simulink library "base_lib"  (R2020b)
settings: Solver=VariableStepAuto  StartTime=0.0  StopTime=10.0  RelTol=1e-3
(part 1 of 2)
settings Model: Creator=maxjo65  LastModifiedBy=Max

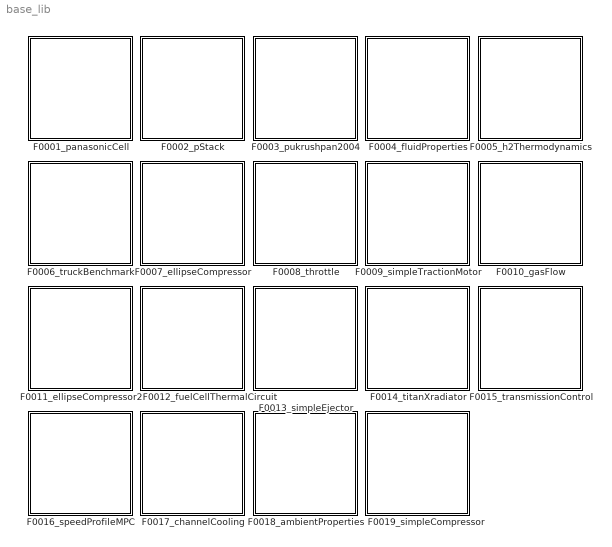
== system base_lib ==
  F0001_panasonicCell : Subsystem
  F0002_pStack : Subsystem
  F0003_pukrushpan2004 : Subsystem
  F0004_fluidProperties : Subsystem
  F0005_h2Thermodynamics : Subsystem
  F0006_truckBenchmark : Subsystem
  F0007_ellipseCompressor : Subsystem
  F0008_throttle : Subsystem
  F0009_simpleTractionMotor : Subsystem
  F0010_gasFlow : Subsystem
  F0011_ellipseCompressor2 : Subsystem
  F0012_fuelCellThermalCircuit : Subsystem
  F0013_simpleEjector : Subsystem
  F0014_titanXradiator : Subsystem
  F0015_transmissionControl : Subsystem
  F0016_speedProfileMPC : Subsystem
  F0017_channelCooling : Subsystem
  F0018_ambientProperties : Subsystem
  F0019_simpleCompressor : Subsystem

== system base_lib/F0001_panasonicCell ==
  F0001_cellCapacity.m : MATLAB Function  TreatAsAtomicUnit=on
  F0001_dynamicVoltage.m : MATLAB Function  TreatAsAtomicUnit=on
  F0001_ocvSOC.m : MATLAB Function  TreatAsAtomicUnit=on

== system base_lib/F0002_pStack ==
  F0002_pStackVoltage.m : MATLAB Function  TreatAsAtomicUnit=on

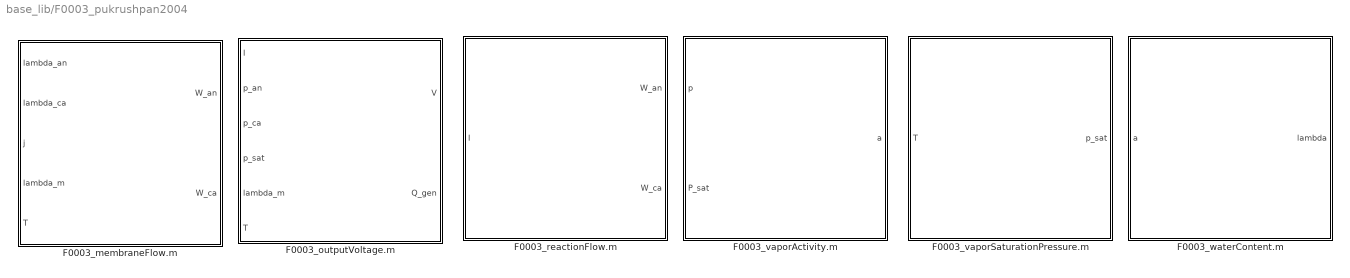
== system base_lib/F0003_pukrushpan2004 ==
  F0003_membraneFlow.m : MATLAB Function  TreatAsAtomicUnit=on
  F0003_outputVoltage.m : MATLAB Function  TreatAsAtomicUnit=on
  F0003_reactionFlow.m : MATLAB Function  TreatAsAtomicUnit=on
  F0003_vaporActivity.m : MATLAB Function  TreatAsAtomicUnit=on
  F0003_vaporSaturationPressure.m : MATLAB Function  TreatAsAtomicUnit=on
  F0003_waterContent.m : MATLAB Function  TreatAsAtomicUnit=on

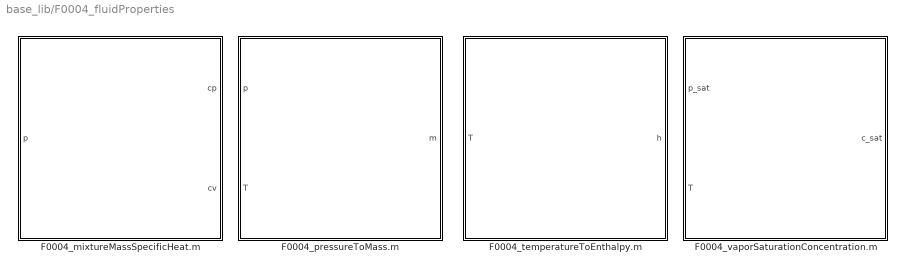
== system base_lib/F0004_fluidProperties ==
  F0004_mixtureMassSpecificHeat.m : MATLAB Function  TreatAsAtomicUnit=on
  F0004_pressureToMass.m : MATLAB Function  TreatAsAtomicUnit=on
  F0004_temperatureToEnthalpy.m : MATLAB Function  TreatAsAtomicUnit=on
  F0004_vaporSaturationConcentration.m : MATLAB Function  TreatAsAtomicUnit=on

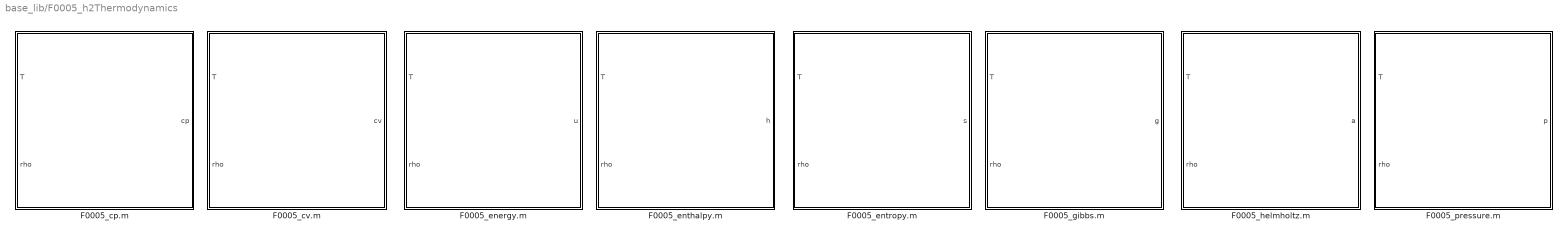
== system base_lib/F0005_h2Thermodynamics ==
  F0005_cp.m : MATLAB Function  TreatAsAtomicUnit=on
  F0005_cv.m : MATLAB Function  TreatAsAtomicUnit=on
  F0005_energy.m : MATLAB Function  TreatAsAtomicUnit=on
  F0005_enthalpy.m : MATLAB Function  TreatAsAtomicUnit=on
  F0005_entropy.m : MATLAB Function  TreatAsAtomicUnit=on
  F0005_gibbs.m : MATLAB Function  TreatAsAtomicUnit=on
  F0005_helmholtz.m : MATLAB Function  TreatAsAtomicUnit=on
  F0005_pressure.m : MATLAB Function  TreatAsAtomicUnit=on

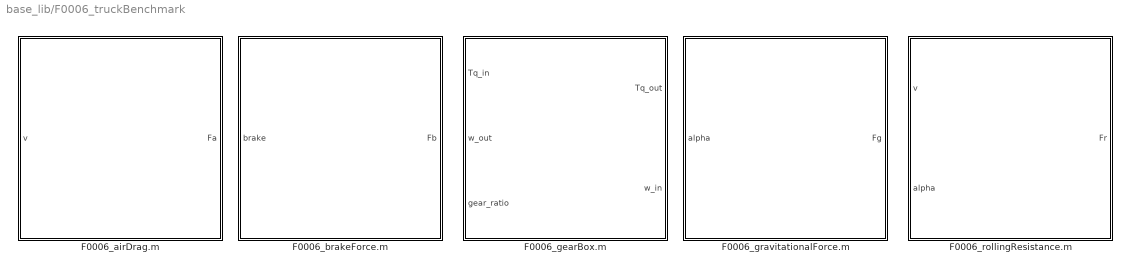
== system base_lib/F0006_truckBenchmark ==
  F0006_airDrag.m : MATLAB Function  TreatAsAtomicUnit=on
  F0006_brakeForce.m : MATLAB Function  TreatAsAtomicUnit=on
  F0006_gearBox.m : MATLAB Function  TreatAsAtomicUnit=on
  F0006_gravitationalForce.m : MATLAB Function  TreatAsAtomicUnit=on
  F0006_rollingResistance.m : MATLAB Function  TreatAsAtomicUnit=on

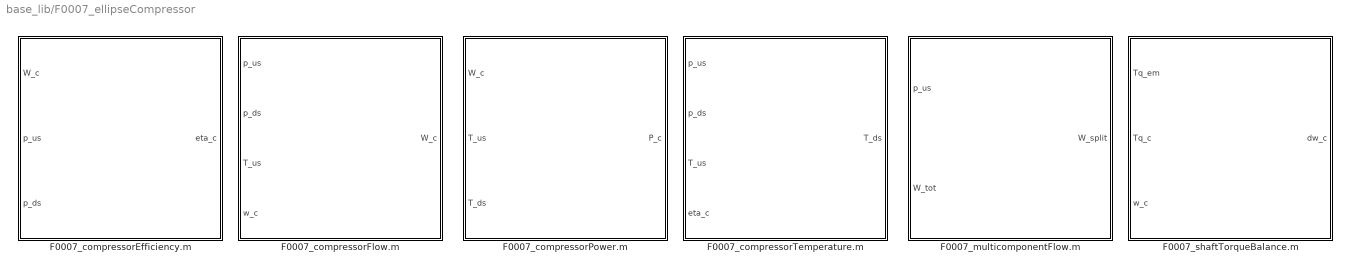
== system base_lib/F0007_ellipseCompressor ==
  F0007_compressorEfficiency.m : MATLAB Function  TreatAsAtomicUnit=on
  F0007_compressorFlow.m : MATLAB Function  TreatAsAtomicUnit=on
  F0007_compressorPower.m : MATLAB Function  TreatAsAtomicUnit=on
  F0007_compressorTemperature.m : MATLAB Function  TreatAsAtomicUnit=on
  F0007_multicomponentFlow.m : MATLAB Function  TreatAsAtomicUnit=on
  F0007_shaftTorqueBalance.m : MATLAB Function  TreatAsAtomicUnit=on

== system base_lib/F0008_throttle ==
  F0008_throttleFlow.m : MATLAB Function  TreatAsAtomicUnit=on
  F0008_throttleFlow2.m : MATLAB Function  TreatAsAtomicUnit=on

== system base_lib/F0009_simpleTractionMotor ==
  F0009_currentDemand.m : MATLAB Function  TreatAsAtomicUnit=on
  F0009_torqueLimit.m : MATLAB Function  TreatAsAtomicUnit=on

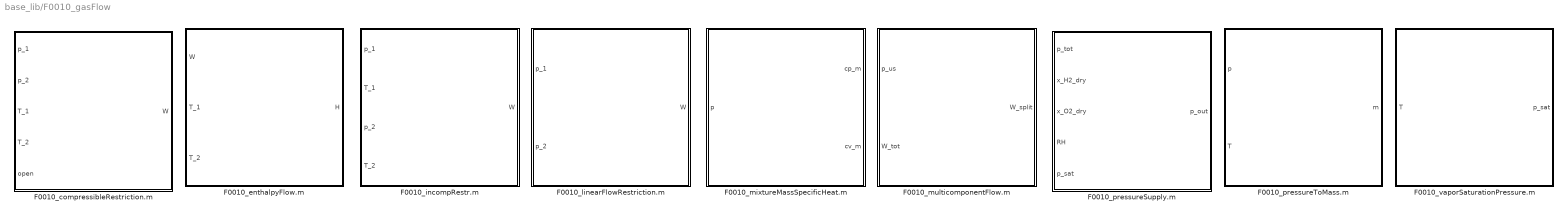
== system base_lib/F0010_gasFlow ==
  F0010_compressibleRestriction.m : MATLAB Function  TreatAsAtomicUnit=on
  F0010_enthalpyFlow.m : MATLAB Function  TreatAsAtomicUnit=on
  F0010_incompRestr.m : MATLAB Function  TreatAsAtomicUnit=on
  F0010_linearFlowRestriction.m : MATLAB Function  TreatAsAtomicUnit=on
  F0010_mixtureMassSpecificHeat.m : MATLAB Function  TreatAsAtomicUnit=on
  F0010_multicomponentFlow.m : MATLAB Function  TreatAsAtomicUnit=on
  F0010_pressureSupply.m : MATLAB Function  TreatAsAtomicUnit=on
  F0010_pressureToMass.m : MATLAB Function  TreatAsAtomicUnit=on
  F0010_vaporSaturationPressure.m : MATLAB Function  TreatAsAtomicUnit=on

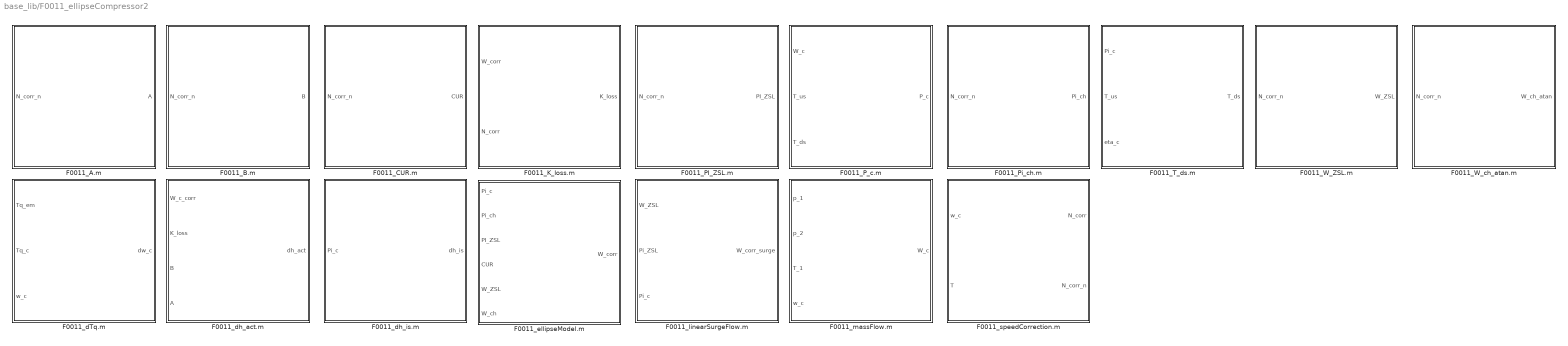
== system base_lib/F0011_ellipseCompressor2 ==
  F0011_A.m : MATLAB Function  TreatAsAtomicUnit=on
  F0011_B.m : MATLAB Function  TreatAsAtomicUnit=on
  F0011_CUR.m : MATLAB Function  TreatAsAtomicUnit=on
  F0011_K_loss.m : MATLAB Function  TreatAsAtomicUnit=on
  F0011_PI_ZSL.m : MATLAB Function  TreatAsAtomicUnit=on
  F0011_P_c.m : MATLAB Function  TreatAsAtomicUnit=on
  F0011_Pi_ch.m : MATLAB Function  TreatAsAtomicUnit=on
  F0011_T_ds.m : MATLAB Function  TreatAsAtomicUnit=on
  F0011_W_ZSL.m : MATLAB Function  TreatAsAtomicUnit=on
  F0011_W_ch_atan.m : MATLAB Function  TreatAsAtomicUnit=on
  F0011_dTq.m : MATLAB Function  TreatAsAtomicUnit=on
  F0011_dh_act.m : MATLAB Function  TreatAsAtomicUnit=on
  F0011_dh_is.m : MATLAB Function  TreatAsAtomicUnit=on
  F0011_ellipseModel.m : MATLAB Function  TreatAsAtomicUnit=on
  F0011_linearSurgeFlow.m : MATLAB Function  TreatAsAtomicUnit=on
  F0011_massFlow.m : MATLAB Function  TreatAsAtomicUnit=on
  F0011_speedCorrection.m : MATLAB Function  TreatAsAtomicUnit=on

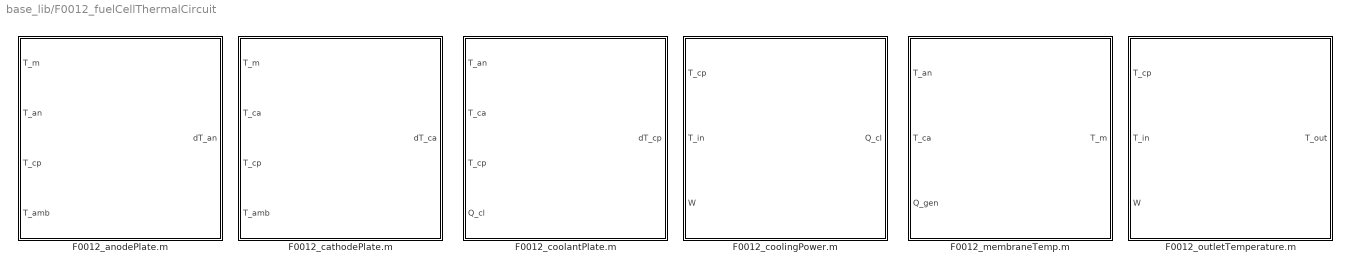
== system base_lib/F0012_fuelCellThermalCircuit ==
  F0012_anodePlate.m : MATLAB Function  TreatAsAtomicUnit=on
  F0012_cathodePlate.m : MATLAB Function  TreatAsAtomicUnit=on
  F0012_coolantPlate.m : MATLAB Function  TreatAsAtomicUnit=on
  F0012_coolingPower.m : MATLAB Function  TreatAsAtomicUnit=on
  F0012_membraneTemp.m : MATLAB Function  TreatAsAtomicUnit=on
  F0012_outletTemperature.m : MATLAB Function  TreatAsAtomicUnit=on

== system base_lib/F0013_simpleEjector ==
  F0013_ejectorModel.m : MATLAB Function  TreatAsAtomicUnit=on

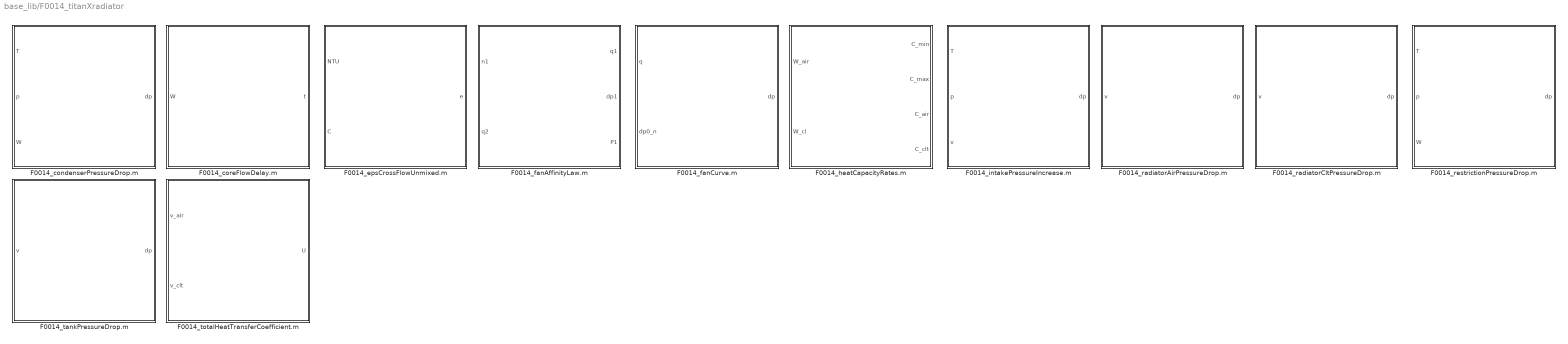
== system base_lib/F0014_titanXradiator ==
  F0014_condenserPressureDrop.m : MATLAB Function  TreatAsAtomicUnit=on
  F0014_coreFlowDelay.m : MATLAB Function  TreatAsAtomicUnit=on
  F0014_epsCrossFlowUnmixed.m : MATLAB Function  TreatAsAtomicUnit=on
  F0014_fanAffinityLaw.m : MATLAB Function  TreatAsAtomicUnit=on
  F0014_fanCurve.m : MATLAB Function  TreatAsAtomicUnit=on
  F0014_heatCapacityRates.m : MATLAB Function  TreatAsAtomicUnit=on
  F0014_intakePressureIncrease.m : MATLAB Function  TreatAsAtomicUnit=on
  F0014_radiatorAirPressureDrop.m : MATLAB Function  TreatAsAtomicUnit=on
  F0014_radiatorCltPressureDrop.m : MATLAB Function  TreatAsAtomicUnit=on
  F0014_restrictionPressureDrop.m : MATLAB Function  TreatAsAtomicUnit=on
  F0014_tankPressureDrop.m : MATLAB Function  TreatAsAtomicUnit=on
  F0014_totalHeatTransferCoefficient.m : MATLAB Function  TreatAsAtomicUnit=on

== system base_lib/F0015_transmissionControl ==
  F0015_gearSelector.m : MATLAB Function  TreatAsAtomicUnit=on
  F0015_transmissionControlUnit.m : MATLAB Function  TreatAsAtomicUnit=on

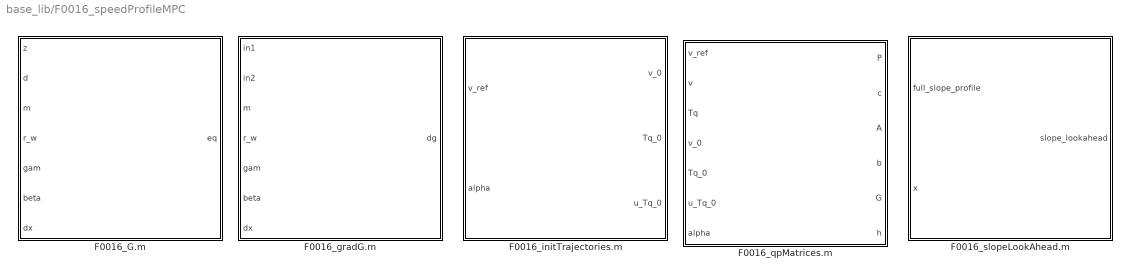
== system base_lib/F0016_speedProfileMPC ==
  F0016_G.m : MATLAB Function  TreatAsAtomicUnit=on
  F0016_gradG.m : MATLAB Function  TreatAsAtomicUnit=on
  F0016_initTrajectories.m : MATLAB Function  TreatAsAtomicUnit=on
  F0016_qpMatrices.m : MATLAB Function  TreatAsAtomicUnit=on
  F0016_slopeLookAhead.m : MATLAB Function  TreatAsAtomicUnit=on

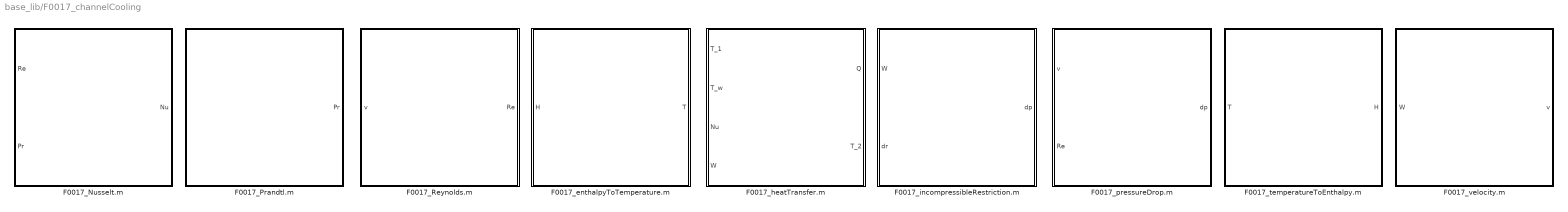
== system base_lib/F0017_channelCooling ==
  F0017_Nusselt.m : MATLAB Function  TreatAsAtomicUnit=on
  F0017_Prandtl.m : MATLAB Function  TreatAsAtomicUnit=on
  F0017_Reynolds.m : MATLAB Function  TreatAsAtomicUnit=on
  F0017_enthalpyToTemperature.m : MATLAB Function  TreatAsAtomicUnit=on
  F0017_heatTransfer.m : MATLAB Function  TreatAsAtomicUnit=on
  F0017_incompressibleRestriction.m : MATLAB Function  TreatAsAtomicUnit=on
  F0017_pressureDrop.m : MATLAB Function  TreatAsAtomicUnit=on
  F0017_temperatureToEnthalpy.m : MATLAB Function  TreatAsAtomicUnit=on
  F0017_velocity.m : MATLAB Function  TreatAsAtomicUnit=on

== system base_lib/F0018_ambientProperties ==
  F0018_troposphereModel.m : MATLAB Function  TreatAsAtomicUnit=on

== system base_lib/F0019_simpleCompressor ==
  F0007_compressorPower.m : MATLAB Function  TreatAsAtomicUnit=on
  F0007_compressorTemperature.m : MATLAB Function  TreatAsAtomicUnit=on
  F0007_multicomponentFlow.m : MATLAB Function  TreatAsAtomicUnit=on

== matlab function base_lib/F0003_pukrushpan2004/F0003_waterContent.m ==
  data: a input; lambda output
function lambda = F0003_waterContent(a)
lambda = zeros(length(a),1);
lambda( a <= 1) = 0.043 + 17.81.*a - 39.85.*a.^2 + 36.*a.^3;
lambda( a > 1)  = 14 + 1.4*(a-1);
end

== matlab function base_lib/F0004_fluidProperties/F0004_mixtureMassSpecificHeat.m ==
  data: p input; cp output; cv output; par parameter
function [cp, cv] = F0004_mixtureMassSpecificHeat(p, par)
% total pressure
p_tot = sum(p);

% mass specific heat capacity
cp_r  = par.cp_r;
cp_v  = par.cp_H2O;
cp_N2 = par.cp_N2;
R_r    = par.R_r;
R_H2O  = par.R_H2O;
R_N2   = par.R_N2;

% partial pressures
p_r  = p(1);
p_v  = p(2);
p_N2 = p(3);

% mole fractions
x_r   = p_r  ./ p_tot;
x_v   = p_v  ./ p_tot;
x_N2  = p_N2 ./ p_tot;

% average mass
M_avg = sum([x_r, x_v, x_N2] .* [par.M_r, par.M_H2O, par.M_N2]);

% mole fraction to mass fraction
w_r   = x_r  .* par.M_r   ./ M_avg;
w_v   = x_v  .* par.M_H2O ./ M_avg;
w_N2  = x_N2 .* par.M_N2  ./ M_avg;

% mixture gas constant
Rm = w_r.*R_r + w_v.*R_H2O + w_N2 .* R_N2;

% ideal mixture heat capacity
cp = w_r.*cp_r + w_v.*cp_v + w_N2 .* cp_N2;
cv = cp - Rm;

end

== matlab function base_lib/F0004_fluidProperties/F0004_pressureToMass.m ==
  data: p input; m output; T input; par parameter
function m = F0004_pressureToMass(p, T, par)
% gas constants
R_r    = par.R_r;
R_H2O  = par.R_H2O;
R_N2   = par.R_N2;
Rj     = [R_r; R_H2O; R_N2];
V      = par.V;

% mass
m = p .* V ./ (Rj .* T);
end

== matlab function base_lib/F0004_fluidProperties/F0004_temperatureToEnthalpy.m ==
  data: T input; h output; par parameter
function h = F0004_temperatureToEnthalpy(T, par)
% output size
h = zeros(3,1);

% mass heat capacity
cp_r  = par.cp_r;
cp_v  = par.cp_H2O;
cp_N2 = par.cp_N2;
cp    = [cp_r; cp_v; cp_N2];

% specific enthalpy
h = cp .* T;
end

== matlab function base_lib/F0004_fluidProperties/F0004_vaporSaturationConcentration.m ==
  data: p_sat input; c_sat output; T input; par parameter
function c_sat = F0004_vaporSaturationConcentration(p_sat, T, par)
% saturation concentration
c_sat = p_sat ./ (par.R .* T);

end

== matlab function base_lib/F0005_h2Thermodynamics/F0005_cp.m ==
  data: T input; cp output; rho input
function cp = F0005_cp(T,rho)
%ISOBARICHEATCAPACITY
%    CP = ISOBARICHEATCAPACITY(T,RHO)

%    This function was generated by the Symbolic Math Toolbox version 8.7.
%    04-Nov-2021 19:06:05

t2 = rho.^2;
t3 = rho.^3;
t4 = 1.0./T;
t5 = rho./1.5508e+4;
t9 = rho.*2.17307196285788e-4;
t10 = rho.*1.328346659788496e-5;
t11 = rho.*6.30642249161723e-5;
t12 = rho.*3.231880319834924e-4;
t13 = rho.*2.072478720660304e-4;
t6 = -t5;
t8 = t4.*3.3145e+1;
t14 = t5-3.9e+1./2.5e+2;
t15 = t5-6.7e+1./1.0e+2;
t16 = t5-2.17e+2./1.25e+2;
t17 = t4.*8.644216;
t18 = t4.*1.133559e+1;
t19 = t4.*1.4882105e+1;
t20 = t4.*1.8461765e+1;
t21 = t5-7.53e+2./5.0e+2;
t22 = t5-8.31e+2./5.0e+2;
t26 = t4.*2.6297243e+1;
t53 = t10-3.57616e-1;
t59 = t9-5.07522;
t60 = t11-1.52568e-1;
t61 = t12-3.35804;
t68 = t13-5.341668;
t69 = t3.*t4.*3.554762889834598e-13;
t92 = t4.*6.858999999999336e+3;
t94 = t4.*5.309999999993605e+2;
t95 = t4.*1.98899999999884e+3;
t97 = t4.*2.484000000001446e+3;
t98 = t4.*7.51000000000887e+2;
t7 = exp(t6);
t23 = t14.^2;
t24 = t15.^2;
t25 = t16.^2;
t27 = t8.^(3.77e+2./5.0e+2);
t28 = t21.^2;
t29 = t22.^2;
t30 = t8.^(3.11e+2./1.0e+3);
t31 = t8.^(8.77e+2./5.0e+2);
t32 = t8.^(4.89e+2./1.0e+3);
t33 = t8.^(9.93e+2./5.0e+2);
t34 = t8.^2.986;
t35 = t8.^4.646;
t36 = t8.^5.646;
t37 = 1.0./t8.^(2.09e+2./1.0e+3);
t38 = t8.^(7.91e+2./1.0e+3);
t39 = t8.^(8.03e+2./1.0e+3);
t40 = t8.^(9.89e+2./1.0e+3);
t41 = t8.^1.311;
t42 = t8.^1.409;
t43 = t8.^3.187;
t44 = t8.^6.844e-1;
t45 = t8.^4.187;
t46 = t8.^1.1444;
t47 = t8.^6.249;
t48 = t8.^7.249;
t49 = t8-7.164e-1;
t50 = t8-7.204e-1;
t51 = t8-1.5445;
t52 = t8-1.3444;
t54 = t8-1.4517;
t77 = t18-2.450088e-1;
t82 = t19-6.036356e-1;
t83 = t20-4.012628e-1;
t84 = t17-3.7860336e-1;
t90 = t26-1.2254063;
t96 = -t92;
t99 = -t94;
t100 = -t95;
t101 = -t97;
t102 = -t98;
t55 = t49.^2;
t56 = t50.^2;
t57 = t51.^2;
t58 = t52.^2;
t62 = t54.^2;
t63 = t23.*(4.89e+2./1.0e+3);
t64 = t25.*(1.03e+2./1.0e+3);
t66 = t28.*(3.37e+2./2.0e+2);
t67 = t24.*2.506;
t73 = t29.*1.607;
t78 = t40.*2.1101;
t91 = rho.*t46.*1.729249419654372e-4;
t103 = exp(t96);
t104 = exp(t99);
t105 = exp(t100);
t106 = exp(t101);
t107 = exp(t102);
t113 = t32.*4.52059;
t114 = t44.*6.93643;
t116 = rho.*t39.*9.447562548362136e-5;
t119 = t7.*t31.*7.77414e-1;
t126 = t2.*t42.*1.633921676808176e-9;
t129 = rho.*t7.*t31.*5.012986845499098e-5;
t131 = t2.*t7.*t41.*4.390189186720438e-9;
t132 = t3.*t7.*t41.*9.43639666993474e-14;
t65 = -t63;
t70 = -t64;
t71 = -t66;
t72 = -t67;
t74 = -t73;
t75 = t55.*(1.71e+2./1.0e+3);
t76 = t58.*2.245e-1;
t80 = t56.*2.785e-1;
t86 = t57.*3.967e-1;
t87 = t62.*1.304e-1;
t93 = -t91;
t108 = t103-1.0;
t109 = t104-1.0;
t110 = t105-1.0;
t111 = t106-1.0;
t112 = t107-1.0;
t115 = -t114;
t122 = -t119;
t133 = -t132;
t79 = -t75;
t81 = -t76;
t85 = -t80;
t88 = -t86;
t89 = -t87;
t117 = t65+t81;
t118 = t71+t79;
t121 = t72+t85;
t124 = t70+t89;
t128 = t74+t88;
t120 = exp(t117);
t123 = exp(t118);
t125 = exp(t121);
t127 = exp(t124);
t130 = exp(t128);
t134 = t36.*t120.*2.26312e-2;
t135 = t48.*t125.*2.31752e-2;
t137 = t34.*t130.*5.57346e-2;
t138 = rho.*t45.*t123.*2.730410110910498e-6;
t140 = t2.*t38.*t127.*4.015042715686892e-10;
t141 = rho.*t36.*t60.*t120.*1.459324219757545e-6;
t143 = rho.*t48.*t61.*t125.*1.494402888831571e-6;
t144 = rho.*t34.*t68.*t130.*3.593925715759608e-6;
t145 = t2.*t45.*t59.*t123.*8.803230948254119e-11;
t147 = t3.*t38.*t53.*t127.*8.630046246425269e-15;
t136 = -t135;
t139 = -t138;
t142 = -t141;
t146 = -t144;
t148 = -t147;
t149 = t69+t78+t93+t113+t115+t116+t122+t126+t129+t131+t133+t134+t136+t137+t139+t140+t142+t143+t145+t146+t148;
et1 = 1.0./t109.^2.*exp(t4.*(-1.061999999998721e+3)).*4.147575991701757e+2;
et2 = 1.0./t110.^2.*exp(t4.*(-3.977999999997681e+3)).*(-2.852060285124163e+3);
et3 = 1.0./t108.^2.*exp(t4.*(-1.371799999999867e+4)).*5.211660743085801e+4;
et4 = 1.0./t111.^2.*exp(t4.*(-4.968000000002893e+3)).*4.257320460091549e+3;
et5 = 1.0./t112.^2.*exp(t4.*(-1.502000000001774e+3)).*(-2.113609217775546e+2)+rho.*1.0./t8.^1.011.*1.480253927005417e-6;
et6 = rho.*1.0./t8.^1.511.*7.283985740327573e-5-rho.*1.0./t8.^1.3156.*9.661114093340211e-5-(t103.*5.211660743085801e+4)./t108;
et7 = (t104.*(-4.147575991701757e+2))./t109+(t105.*2.852060285124163e+3)./t110;
et8 = (t106.*(-4.257320460091549e+3))./t111+(t107.*2.113609217775546e+2)./t112;
et9 = t3.*1.0./t8.^(5.91e+2./1.0e+3).*(-2.023897381636773e-14)+t2.*1.0./t8.^1.197.*4.818543226360442e-10+t2.*1.0./t8.^8.556e-1.*9.213335645379665e-10;
et10 = 1.0./t4.^2.*1.365385267005982e-3+rho.*t7.*1.0./t8.^(1.23e+2./5.0e+2).*6.629755310962085e-5-rho.*t8.^(4.93e+2./5.0e+2).*t130.*2.131268390389476e-5;
et11 = rho.*t8.^3.646.*t120.*(-3.827999475491359e-5)+rho.*t8.^5.249.*t125.*6.769495795558421e-5;
et12 = t3.*t7.*1.0./t8.^(6.89e+2./1.0e+3).*(-3.847417086662462e-14)+t3.*1.0./t8.^1.209.*t127.*1.426710615412779e-15;
et13 = t2.*t8.^2.187.*t123.*1.174700408733436e-9+rho.*t36.*t120.*6.552365746711375e-7+rho.*t34.*t130.*2.851420662883673e-6;
et14 = rho.*t48.*t125.*(-8.323824090791849e-7)+t3.*t38.*t127.*2.25071606106771e-15-t2.*t45.*t123.*3.010704984302909e-11;
et15 = rho.*t35.*t82.*t120.*1.647868908950219e-5+rho.*t33.*t90.*t130.*2.146292437451638e-5-rho.*t47.*t83.*t125.*2.166585308228011e-5;
et16 = t2.*t43.*t77.*t123.*(-7.371825596068e-10)+t3.*t37.*t84.*t127.*1.365273316184478e-14-rho.*t36.*t82.^2.*t120.*1.459324219757545e-6;
et17 = rho.*t34.*t90.^2.*t130.*(-3.593925715759608e-6)+rho.*t48.*t83.^2.*t125.*1.494402888831571e-6+t2.*t45.*t77.^2.*t123.*8.803230948254119e-11-t3.*t38.*t84.^2.*t127.*8.630046246425269e-15;
et18 = t39.*1.465128-t46.*2.68172-t129+t132+rho.*t42.*5.067771472788238e-5+t2.*t4.*1.653817886866649e-8+t7.*t31.*1.554828-t45.*t123.*4.23432e-2+t53.*t147+t60.*t141+t68.*t144;
et19 = rho.*t7.*t41.*1.361661078153211e-4-rho.*t36.*t120.*1.427219086922879e-6-rho.*t34.*t130.*1.155087725045138e-5+rho.*t38.*t127.*1.245305648697446e-5;
et20 = rho.*t48.*t125.*7.489947278823833e-6-t2.*t7.*t41.*8.780378373440877e-9-t3.*t38.*t127.*1.777789526763605e-15;
et21 = t2.*t45.*t123.*2.966688829561638e-10-t36.*t60.*t120.*4.52624e-2-t34.*t68.*t130.*1.114692e-1+t48.*t61.*t125.*4.63504e-2;
et22 = rho.*t45.*t59.*t123.*5.460820221820995e-6-t2.*t38.*t53.*t127.*8.030085431373784e-10-rho.*t48.*t61.^2.*t125.*1.494402888831571e-6-t2.*t45.*t59.^2.*t123.*8.803230948254119e-11;
et23 = t3./9.32410994128e+13-t7.*t27.*1.363584156+t35.*t120.*1.277757552e-1+t33.*t130.*1.664235156e-1-t47.*t125.*1.679970248e-1+t77.*t138+t83.*t135;
et24 = t82.*t141+t84.*t147+t90.*t144+rho.*1.0./t8.^(1.97e+2./1.0e+3).*7.586392726334795e-5-rho.*t8.^1.444e-1.*1.978953035852463e-4+t2.*t8.^(4.09e+2./1.0e+3).*2.30219564262272e-9+1.0./t8.^(1.1e+1./1.0e+3).*2.0868889;
et25 = 1.0./t8.^(5.11e+2./1.0e+3).*2.21056851-1.0./t8.^3.156e-1.*4.747292692+rho.*t7.*t27.*8.792778927005417e-5-rho.*t43.*t123.*1.143222713438225e-5;
et26 = t2.*t7.*t30.*5.755538023790495e-9-t3.*t7.*t30.*1.237111603428444e-13+t2.*t37.*t127.*3.175898788108332e-10;
et27 = t36.*t82.*t120.*(-2.26312e-2)-t34.*t90.*t130.*5.57346e-2-rho.*t35.*t60.*t120.*8.239344544751096e-6-rho.*t33.*t68.*t130.*1.073146218725819e-5;
et28 = rho.*t47.*t61.*t125.*1.083292654114006e-5-t3.*t37.*t53.*t127.*6.826366580922388e-15+t2.*t43.*t59.*t123.*3.685912798034e-10;
et29 = t2.*t38.*t84.*t127.*(-4.015042715686892e-10)-rho.*t48.*t61.*t83.*t125.*1.494402888831571e-6-t2.*t45.*t59.*t77.*t123.*8.803230948254119e-11;
cp = ((t5.*t149-rho.*t4.*(et23+et24+et25+et26+et27+et28+et29).*2.137283982460665e-3+1.0).^2.*8.314472)./((t2.*(et18+et19+et20+et21+et22))./2.40498064e+8+(rho.*t149)./7.754e+3+1.0)+t4.^2.*(et1+et2+et3+et4+et5+et6+et7+et8+et9+et10+et11+et12+et13+et14+et15+et16+et17).*9.1342043168138e+3;

== matlab function base_lib/F0005_h2Thermodynamics/F0005_cv.m ==
  data: T input; cv output; rho input
function cv = F0005_cv(T,rho)
%ISOCHORICHEATCAPACITY
%    CV = ISOCHORICHEATCAPACITY(T,RHO)

%    This function was generated by the Symbolic Math Toolbox version 8.7.
%    04-Nov-2021 19:06:04

t2 = rho.^2;
t3 = rho.^3;
t4 = 1.0./T;
t5 = rho./1.5508e+4;
t6 = -t5;
t8 = t4.*3.3145e+1;
t9 = t5-3.9e+1./2.5e+2;
t10 = t5-6.7e+1./1.0e+2;
t11 = t5-2.17e+2./1.25e+2;
t12 = t4.*8.644216;
t13 = t4.*1.133559e+1;
t14 = t4.*1.4882105e+1;
t15 = t4.*1.8461765e+1;
t16 = t5-7.53e+2./5.0e+2;
t17 = t5-8.31e+2./5.0e+2;
t21 = t4.*2.6297243e+1;
t64 = t4.*6.858999999999336e+3;
t65 = t4.*5.309999999993605e+2;
t66 = t4.*1.98899999999884e+3;
t68 = t4.*2.484000000001446e+3;
t69 = t4.*7.51000000000887e+2;
t7 = exp(t6);
t18 = t9.^2;
t19 = t10.^2;
t20 = t11.^2;
t22 = t16.^2;
t23 = t17.^2;
t24 = t8.^2.986;
t25 = t8.^5.646;
t26 = t8.^(7.91e+2./1.0e+3);
t27 = t8.^4.187;
t28 = t8.^7.249;
t29 = t8-7.164e-1;
t30 = t8-7.204e-1;
t31 = t8-1.5445;
t32 = t8-1.3444;
t33 = t8-1.4517;
t51 = t13-2.450088e-1;
t55 = t14-6.036356e-1;
t56 = t15-4.012628e-1;
t57 = t12-3.7860336e-1;
t63 = t21-1.2254063;
t67 = -t64;
t70 = -t65;
t71 = -t66;
t72 = -t68;
t73 = -t69;
t34 = t29.^2;
t35 = t30.^2;
t36 = t31.^2;
t37 = t32.^2;
t38 = t33.^2;
t39 = t18.*(4.89e+2./1.0e+3);
t40 = t20.*(1.03e+2./1.0e+3);
t42 = t22.*(3.37e+2./2.0e+2);
t43 = t19.*2.506;
t47 = t23.*1.607;
t74 = exp(t67);
t75 = exp(t70);
t76 = exp(t71);
t77 = exp(t72);
t78 = exp(t73);
t41 = -t39;
t44 = -t40;
t45 = -t42;
t46 = -t43;
t48 = -t47;
t49 = t34.*(1.71e+2./1.0e+3);
t50 = t37.*2.245e-1;
t53 = t35.*2.785e-1;
t59 = t36.*3.967e-1;
t60 = t38.*1.304e-1;
t79 = t74-1.0;
t80 = t75-1.0;
t81 = t76-1.0;
t82 = t77-1.0;
t83 = t78-1.0;
t52 = -t49;
t54 = -t50;
t58 = -t53;
t61 = -t59;
t62 = -t60;
t84 = t41+t54;
t85 = t45+t52;
t87 = t46+t58;
t89 = t44+t62;
t92 = t48+t61;
t86 = exp(t84);
t88 = exp(t85);
t90 = exp(t87);
t91 = exp(t89);
t93 = exp(t92);
et1 = 1.0./t80.^2.*exp(t4.*(-1.061999999998721e+3)).*4.147575991701757e+2;
et2 = 1.0./t81.^2.*exp(t4.*(-3.977999999997681e+3)).*(-2.852060285124163e+3);
et3 = 1.0./t79.^2.*exp(t4.*(-1.371799999999867e+4)).*5.211660743085801e+4;
et4 = 1.0./t82.^2.*exp(t4.*(-4.968000000002893e+3)).*4.257320460091549e+3;
et5 = 1.0./t83.^2.*exp(t4.*(-1.502000000001774e+3)).*(-2.113609217775546e+2)+rho.*1.0./t8.^1.011.*1.480253927005417e-6;
et6 = rho.*1.0./t8.^1.511.*7.283985740327573e-5-rho.*1.0./t8.^1.3156.*9.661114093340211e-5-(t74.*5.211660743085801e+4)./t79;
et7 = (t75.*(-4.147575991701757e+2))./t80+(t76.*2.852060285124163e+3)./t81;
et8 = (t77.*(-4.257320460091549e+3))./t82+(t78.*2.113609217775546e+2)./t83;
et9 = t3.*1.0./t8.^(5.91e+2./1.0e+3).*(-2.023897381636773e-14)+t2.*1.0./t8.^1.197.*4.818543226360442e-10+t2.*1.0./t8.^8.556e-1.*9.213335645379665e-10;
et10 = 1.0./t4.^2.*1.365385267005982e-3+rho.*t7.*1.0./t8.^(1.23e+2./5.0e+2).*6.629755310962085e-5-rho.*t8.^(4.93e+2./5.0e+2).*t93.*2.131268390389476e-5;
et11 = rho.*t8.^3.646.*t86.*(-3.827999475491359e-5)+rho.*t8.^5.249.*t90.*6.769495795558421e-5;
et12 = t3.*t7.*1.0./t8.^(6.89e+2./1.0e+3).*(-3.847417086662462e-14)+t3.*1.0./t8.^1.209.*t91.*1.426710615412779e-15;
et13 = t2.*t8.^2.187.*t88.*1.174700408733436e-9+rho.*t25.*t86.*6.552365746711375e-7+rho.*t24.*t93.*2.851420662883673e-6;
et14 = rho.*t28.*t90.*(-8.323824090791849e-7)-t2.*t27.*t88.*3.010704984302909e-11+t3.*t26.*t91.*2.25071606106771e-15;
et15 = rho.*t25.*t55.^2.*t86.*(-1.459324219757545e-6)+rho.*t28.*t56.^2.*t90.*1.494402888831571e-6-rho.*t24.*t63.^2.*t93.*3.593925715759608e-6+rho.*t8.^(9.93e+2./5.0e+2).*t63.*t93.*2.146292437451638e-5;
et16 = rho.*t8.^4.646.*t55.*t86.*1.647868908950219e-5-rho.*t8.^6.249.*t56.*t90.*2.166585308228011e-5+t2.*t27.*t51.^2.*t88.*8.803230948254119e-11;
et17 = t3.*t26.*t57.^2.*t91.*(-8.630046246425269e-15)+t3.*1.0./t8.^(2.09e+2./1.0e+3).*t57.*t91.*1.365273316184478e-14-t2.*t8.^3.187.*t51.*t88.*7.371825596068e-10;
cv = t4.^2.*(et1+et2+et3+et4+et5+et6+et7+et8+et9+et10+et11+et12+et13+et14+et15+et16+et17).*9.1342043168138e+3;

== matlab function base_lib/F0005_h2Thermodynamics/F0005_energy.m ==
  data: T input; u output; rho input
function u = F0005_energy(T,rho)
%INTERNALENERGY
%    U = INTERNALENERGY(T,RHO)

%    This function was generated by the Symbolic Math Toolbox version 8.7.
%    04-Nov-2021 19:06:03

t2 = rho.^2;
t3 = rho.^3;
t4 = 1.0./T;
t5 = rho./1.5508e+4;
t6 = -t5;
t8 = t4.*3.3145e+1;
t9 = t5-3.9e+1./2.5e+2;
t10 = t5-6.7e+1./1.0e+2;
t11 = t5-2.17e+2./1.25e+2;
t12 = t5-7.53e+2./5.0e+2;
t13 = t5-8.31e+2./5.0e+2;
t49 = t4.*6.858999999999336e+3;
t50 = t4.*5.309999999993605e+2;
t51 = t4.*1.98899999999884e+3;
t53 = t4.*2.484000000001446e+3;
t54 = t4.*7.51000000000887e+2;
t7 = exp(t6);
t14 = t9.^2;
t15 = t10.^2;
t16 = t11.^2;
t17 = t12.^2;
t18 = t13.^2;
t19 = t8-7.164e-1;
t20 = t8-7.204e-1;
t21 = t8-1.5445;
t22 = t8-1.3444;
t23 = t8-1.4517;
t52 = -t49;
t55 = -t50;
t56 = -t51;
t57 = -t53;
t58 = -t54;
t24 = t19.^2;
t25 = t20.^2;
t26 = t21.^2;
t27 = t22.^2;
t28 = t23.^2;
t29 = t14.*(4.89e+2./1.0e+3);
t30 = t16.*(1.03e+2./1.0e+3);
t32 = t17.*(3.37e+2./2.0e+2);
t33 = t15.*2.506;
t37 = t18.*1.607;
t59 = exp(t52);
t60 = exp(t55);
t61 = exp(t56);
t62 = exp(t57);
t63 = exp(t58);
t31 = -t29;
t34 = -t30;
t35 = -t32;
t36 = -t33;
t38 = -t37;
t39 = t24.*(1.71e+2./1.0e+3);
t40 = t27.*2.245e-1;
t42 = t25.*2.785e-1;
t45 = t26.*3.967e-1;
t46 = t28.*1.304e-1;
t41 = -t39;
t43 = -t40;
t44 = -t42;
t47 = -t45;
t48 = -t46;
t64 = t31+t43;
t65 = t35+t41;
t67 = t36+t44;
t69 = t34+t48;
t72 = t38+t47;
t66 = exp(t64);
t68 = exp(t65);
t70 = exp(t67);
t71 = exp(t69);
t73 = exp(t72);
et1 = T.*1.2471708e+1-(t59.*6.940424851620928e+4)./(t59-1.0);
et2 = (t60.*(-7.134615165303407e+3))./(t60-1.0)+(t61.*1.309768796792836e+4)./(t61-1.0);
et3 = (t62.*(-1.565508652359312e+4))./(t62-1.0)+(t63.*2.570724159925436e+3)./(t63-1.0);
et4 = rho.*1.0./t8.^(1.1e+1./1.0e+3).*3.708482510740261e-2+rho.*1.0./t8.^(5.11e+2./1.0e+3).*3.928265974354533e-2;
et5 = rho.*1.0./t8.^3.156e-1.*(-8.436123227090361e-2)+t2.*1.0./t8.^(1.97e+2./1.0e+3).*6.740657048206955e-7;
et6 = t3.*t8.^(4.09e+2./1.0e+3).*1.363696980861286e-11-t2.*t8.^1.444e-1.*1.758338147046353e-6;
et7 = t2.^2.*4.764633820313524e-17-rho.*t7.*t8.^(3.77e+2./5.0e+2).*2.42314192885329e-2;
et8 = rho.*t8.^(9.93e+2./5.0e+2).*t73.*2.957410415947438e-3+rho.*t8.^4.646.*t66.*2.270624724947404e-3;
et9 = rho.*t8.^6.249.*t70.*(-2.985372284682706e-3)+t3.*1.0./t8.^(2.09e+2./1.0e+3).*t71.*1.881231772261721e-12;
et10 = t3.*t7.*t8.^(3.11e+2./1.0e+3).*3.409271428093691e-11;
et11 = t2.*t8.^3.187.*t68.*(-1.015775549591232e-7);
et12 = rho.*t8.^5.646.*t66.*(t4.*1.4882105e+1-6.036356e-1).*(-4.021652010179603e-4);
et13 = rho.*t8.^7.249.*t70.*(t4.*1.8461765e+1-4.012628e-1).*4.118322919965107e-4;
et14 = t2.*t8.^4.187.*t68.*(t4.*1.133559e+1-2.450088e-1).*2.426022330048322e-8;
et15 = t3.*t8.^(7.91e+2./1.0e+3).*t71.*(t4.*8.644216-3.7860336e-1).*(-2.378295540153882e-12);
et16 = rho.*t8.^2.986.*t73.*(t4.*2.6297243e+1-1.2254063).*(-9.90425457450582e-4)+5.203221931700199e+2;
u = et1+et2+et3+et4+et5+et6+et7+et8+et9+et10+et11+et12+et13+et14+et15+et16;

== matlab function base_lib/F0005_h2Thermodynamics/F0005_enthalpy.m ==
  data: T input; h output; rho input
function h = F0005_enthalpy(T,rho)
%ENTHALPY
%    H = ENTHALPY(T,RHO)

%    This function was generated by the Symbolic Math Toolbox version 8.7.
%    04-Nov-2021 19:06:04

t2 = rho.^2;
t3 = rho.^3;
t4 = 1.0./T;
t5 = rho./1.5508e+4;
t6 = -t5;
t8 = t4.*3.3145e+1;
t9 = t5-3.9e+1./2.5e+2;
t10 = t5-6.7e+1./1.0e+2;
t11 = t5-2.17e+2./1.25e+2;
t12 = t5-7.53e+2./5.0e+2;
t13 = t5-8.31e+2./5.0e+2;
t56 = t4.*6.858999999999336e+3;
t57 = t4.*5.309999999993605e+2;
t58 = t4.*1.98899999999884e+3;
t60 = t4.*2.484000000001446e+3;
t61 = t4.*7.51000000000887e+2;
t7 = exp(t6);
t14 = t9.^2;
t15 = t10.^2;
t16 = t11.^2;
t17 = t12.^2;
t18 = t13.^2;
t19 = t8.^(8.77e+2./5.0e+2);
t20 = t8.^2.986;
t21 = t8.^5.646;
t22 = t8.^(7.91e+2./1.0e+3);
t23 = t8.^1.311;
t24 = t8.^4.187;
t25 = t8.^7.249;
t26 = t8-7.164e-1;
t27 = t8-7.204e-1;
t28 = t8-1.5445;
t29 = t8-1.3444;
t30 = t8-1.4517;
t59 = -t56;
t62 = -t57;
t63 = -t58;
t64 = -t60;
t65 = -t61;
t31 = t26.^2;
t32 = t27.^2;
t33 = t28.^2;
t34 = t29.^2;
t35 = t30.^2;
t36 = t14.*(4.89e+2./1.0e+3);
t37 = t16.*(1.03e+2./1.0e+3);
t39 = t17.*(3.37e+2./2.0e+2);
t40 = t15.*2.506;
t44 = t18.*1.607;
t66 = exp(t59);
t67 = exp(t62);
t68 = exp(t63);
t69 = exp(t64);
t70 = exp(t65);
t38 = -t36;
t41 = -t37;
t42 = -t39;
t43 = -t40;
t45 = -t44;
t46 = t31.*(1.71e+2./1.0e+3);
t47 = t34.*2.245e-1;
t49 = t32.*2.785e-1;
t52 = t33.*3.967e-1;
t53 = t35.*1.304e-1;
t48 = -t46;
t50 = -t47;
t51 = -t49;
t54 = -t52;
t55 = -t53;
t71 = t38+t50;
t72 = t42+t48;
t74 = t43+t51;
t76 = t41+t55;
t79 = t45+t54;
t73 = exp(t71);
t75 = exp(t72);
t77 = exp(t74);
t78 = exp(t76);
t80 = exp(t79);
et1 = T.*4.525569467491326e-2-(t66.*2.518450143309456e+2)./(t66-1.0)-(t67.*2.58891537184784e+1)./(t67-1.0)+(t68.*4.75271685020088e+1)./(t68-1.0)-(t69.*5.68071202293286e+1)./(t69-1.0);
et2 = (t70.*9.32830592850702)./(t70-1.0)+rho.*1.0./t8.^(1.1e+1./1.0e+3).*1.345685388186742e-4+rho.*1.0./t8.^(5.11e+2./1.0e+3).*1.425437522568997e-4-rho.*1.0./t8.^3.156e-1.*3.061189509930358e-4;
et3 = t2.*1.0./t8.^(1.97e+2./1.0e+3).*2.445961028609361e-9+t3.*t8.^(4.09e+2./1.0e+3).*4.94840435608013e-14-t2.*t8.^1.444e-1.*6.380426347215835e-9+t2.^2./5.78393187877481e+18;
et4 = rho.*t7.*t8.^(3.77e+2./5.0e+2).*(-8.792778927005417e-5)+rho.*t8.^(9.93e+2./5.0e+2).*t80.*1.073146218725819e-5+rho.*t8.^4.646.*t73.*8.239344544751096e-6;
et5 = rho.*t8.^6.249.*t77.*(-1.083292654114006e-5)+t3.*1.0./t8.^(2.09e+2./1.0e+3).*t78.*6.826366580922388e-15+t3.*t7.*t8.^(3.11e+2./1.0e+3).*1.237111603428444e-13;
et6 = t2.*t8.^3.187.*t75.*(-3.685912798034e-10)-rho.*t21.*t73.*(t4.*1.4882105e+1-6.036356e-1).*1.459324219757545e-6;
et7 = rho.*t25.*t77.*(t4.*1.8461765e+1-4.012628e-1).*1.494402888831571e-6+t2.*t24.*t75.*(t4.*1.133559e+1-2.450088e-1).*8.803230948254119e-11;
et8 = t3.*t22.*t78.*(t4.*8.644216-3.7860336e-1).*(-8.630046246425269e-15)-rho.*t20.*t80.*(t4.*2.6297243e+1-1.2254063).*3.593925715759608e-6+1.888076782;
et9 = t3.*t4.*3.554762889834598e-13-t7.*t19.*7.77414e-1+t21.*t73.*2.26312e-2+t20.*t80.*5.57346e-2-t25.*t77.*2.31752e-2;
et10 = rho.*t8.^(8.03e+2./1.0e+3).*9.447562548362136e-5-rho.*t8.^1.1444.*1.729249419654372e-4+t2.*t8.^1.409.*1.633921676808176e-9+t8.^(4.89e+2./1.0e+3).*4.52059;
et11 = t8.^(9.89e+2./1.0e+3).*2.1101-t8.^6.844e-1.*6.93643+rho.*t7.*t19.*5.012986845499098e-5-rho.*t24.*t75.*2.730410110910498e-6+t2.*t7.*t23.*4.390189186720438e-9;
et12 = t3.*t7.*t23.*(-9.43639666993474e-14)+t2.*t22.*t78.*4.015042715686892e-10+rho.*t25.*t77.*(rho.*3.231880319834924e-4-3.35804).*1.494402888831571e-6;
et13 = rho.*t21.*t73.*(rho.*6.30642249161723e-5-1.52568e-1).*(-1.459324219757545e-6)-rho.*t20.*t80.*(rho.*2.072478720660304e-4-5.341668).*3.593925715759608e-6;
et14 = t2.*t24.*t75.*(rho.*2.17307196285788e-4-5.07522).*8.803230948254119e-11-t3.*t22.*t78.*(rho.*1.328346659788496e-5-3.57616e-1).*8.630046246425269e-15;
h = T.*(t8.*(et1+et2+et3+et4+et5+et6+et7+et8)+t5.*(et9+et10+et11+et12+et13+et14)+1.0).*8.314472;

== matlab function base_lib/F0005_h2Thermodynamics/F0005_entropy.m ==
  data: T input; s output; rho input
function s = F0005_entropy(T,rho)
%ENTROPY
%    S = ENTROPY(T,RHO)

%    This function was generated by the Symbolic Math Toolbox version 8.7.
%    04-Nov-2021 19:06:03

t2 = rho.^2;
t3 = rho.^3;
t5 = 1.0./T;
t6 = rho./1.5508e+4;
t4 = t2.^2;
t7 = -t6;
t9 = t5.*3.3145e+1;
t10 = t6-3.9e+1./2.5e+2;
t11 = t6-6.7e+1./1.0e+2;
t12 = t6-2.17e+2./1.25e+2;
t13 = t6-7.53e+2./5.0e+2;
t14 = t6-8.31e+2./5.0e+2;
t55 = t5.*6.858999999999336e+3;
t56 = t5.*5.309999999993605e+2;
t57 = t5.*1.98899999999884e+3;
t59 = t5.*2.484000000001446e+3;
t60 = t5.*7.51000000000887e+2;
t8 = exp(t7);
t15 = t10.^2;
t16 = t11.^2;
t17 = t12.^2;
t18 = t13.^2;
t19 = t14.^2;
t20 = t9.^2.986;
t21 = t9.^5.646;
t22 = t9.^(7.91e+2./1.0e+3);
t23 = t9.^4.187;
t24 = t9.^7.249;
t25 = t9-7.164e-1;
t26 = t9-7.204e-1;
t27 = t9-1.5445;
t28 = t9-1.3444;
t29 = t9-1.4517;
t58 = -t55;
t61 = -t56;
t62 = -t57;
t63 = -t59;
t64 = -t60;
t30 = t25.^2;
t31 = t26.^2;
t32 = t27.^2;
t33 = t28.^2;
t34 = t29.^2;
t35 = t15.*(4.89e+2./1.0e+3);
t36 = t17.*(1.03e+2./1.0e+3);
t38 = t18.*(3.37e+2./2.0e+2);
t39 = t16.*2.506;
t43 = t19.*1.607;
t65 = exp(t58);
t66 = exp(t61);
t67 = exp(t62);
t68 = exp(t63);
t69 = exp(t64);
t37 = -t35;
t40 = -t36;
t41 = -t38;
t42 = -t39;
t44 = -t43;
t45 = t30.*(1.71e+2./1.0e+3);
t46 = t33.*2.245e-1;
t48 = t31.*2.785e-1;
t51 = t32.*3.967e-1;
t52 = t34.*1.304e-1;
t47 = -t45;
t49 = -t46;
t50 = -t48;
t53 = -t51;
t54 = -t52;
t70 = t37+t49;
t71 = t41+t47;
t73 = t42+t50;
t75 = t40+t54;
t78 = t44+t53;
t72 = exp(t70);
t74 = exp(t71);
t76 = exp(t73);
t77 = exp(t75);
t79 = exp(t78);
et1 = T.*4.525569467491326e-2+t4./5.78393187877481e+18-(t65.*2.518450143309456e+2)./(t65-1.0)-(t66.*2.58891537184784e+1)./(t66-1.0)+(t67.*4.75271685020088e+1)./(t67-1.0);
et2 = (t68.*(-5.68071202293286e+1))./(t68-1.0)+(t69.*9.32830592850702)./(t69-1.0)+rho.*1.0./t9.^(1.1e+1./1.0e+3).*1.345685388186742e-4+rho.*1.0./t9.^(5.11e+2./1.0e+3).*1.425437522568997e-4;
et3 = rho.*1.0./t9.^3.156e-1.*(-3.061189509930358e-4)+t2.*1.0./t9.^(1.97e+2./1.0e+3).*2.445961028609361e-9+t3.*t9.^(4.09e+2./1.0e+3).*4.94840435608013e-14;
et4 = t2.*t9.^1.444e-1.*(-6.380426347215835e-9)-rho.*t8.*t9.^(3.77e+2./5.0e+2).*8.792778927005417e-5+rho.*t9.^(9.93e+2./5.0e+2).*t79.*1.073146218725819e-5;
et5 = rho.*t9.^4.646.*t72.*8.239344544751096e-6-rho.*t9.^6.249.*t76.*1.083292654114006e-5+t3.*1.0./t9.^(2.09e+2./1.0e+3).*t77.*6.826366580922388e-15;
et6 = t3.*t8.*t9.^(3.11e+2./1.0e+3).*1.237111603428444e-13-t2.*t9.^3.187.*t74.*3.685912798034e-10;
et7 = rho.*t21.*t72.*(t5.*1.4882105e+1-6.036356e-1).*(-1.459324219757545e-6)+rho.*t24.*t76.*(t5.*1.8461765e+1-4.012628e-1).*1.494402888831571e-6;
et8 = t2.*t23.*t74.*(t5.*1.133559e+1-2.450088e-1).*8.803230948254119e-11-t3.*t22.*t77.*(t5.*8.644216-3.7860336e-1).*8.630046246425269e-15;
et9 = rho.*t20.*t79.*(t5.*2.6297243e+1-1.2254063).*(-3.593925715759608e-6)+1.888076782;
et10 = t5.*(-5.203221931700199e+2)-log(-t65+1.0).*1.0118712424e+1-log(-t66+1.0).*1.3436186752e+1;
et11 = log(-t67+1.0).*6.585061824-log(-t68+1.0).*6.302369776+log(-t69+1.0).*3.4230681224-log(t6).*8.314472;
et12 = log(t9).*(-1.2471708e+1)-t4.*t5.*4.764633820313524e-17-rho.*t9.^(4.89e+2./1.0e+3).*2.423672877126645e-3;
et13 = rho.*t9.^(9.89e+2./1.0e+3).*(-1.131310766520506e-3)+rho.*t9.^6.844e-1.*3.718903341176167e-3;
et14 = t2.*t9.^(8.03e+2./1.0e+3).*(-2.532612015624375e-8)-t3.*t9.^1.409.*2.920040416132454e-13;
et15 = t2.*t9.^1.1444.*4.635606100313556e-8+t5.*(et1+et2+et3+et4+et5+et6+et7+et8+et9).*2.7558317444e+2+rho.*t8.*t9.^(8.77e+2./5.0e+2).*4.168033876327057e-4;
et16 = t3.*t8.*t9.^1.311.*(-7.845865589306564e-13)-rho.*t21.*t72.*1.213351036409595e-5;
et17 = rho.*t20.*t79.*(-2.988159473376322e-5)+rho.*t24.*t76.*1.242517097590921e-5;
et18 = t2.*t23.*t74.*7.319421722879233e-10-t3.*t22.*t77.*7.1754277874608e-14;
et19 = 1.212238084254062e+1;
s = et10+et11+et12+et13+et14+et15+et16+et17+et18+et19;

== matlab function base_lib/F0005_h2Thermodynamics/F0005_gibbs.m ==
  data: T input; g output; rho input
function g = F0005_gibbs(T,rho)
%GIBBSENERGY
%    G = GIBBSENERGY(T,RHO)

%    This function was generated by the Symbolic Math Toolbox version 8.7.
%    04-Nov-2021 19:06:06

t2 = rho.^2;
t3 = rho.^3;
t4 = 1.0./T;
t5 = rho./1.5508e+4;
t6 = -t5;
t8 = t4.*3.3145e+1;
t9 = t5-3.9e+1./2.5e+2;
t10 = t5-6.7e+1./1.0e+2;
t11 = t5-2.17e+2./1.25e+2;
t12 = t5-7.53e+2./5.0e+2;
t13 = t5-8.31e+2./5.0e+2;
t7 = exp(t6);
t14 = t9.^2;
t15 = t10.^2;
t16 = t11.^2;
t17 = t12.^2;
t18 = t13.^2;
t19 = t8.^(8.77e+2./5.0e+2);
t20 = t8.^(4.89e+2./1.0e+3);
t21 = t8.^2.986;
t22 = t8.^5.646;
t23 = t8.^(7.91e+2./1.0e+3);
t24 = t8.^(8.03e+2./1.0e+3);
t25 = t8.^(9.89e+2./1.0e+3);
t26 = t8.^1.311;
t27 = t8.^1.409;
t28 = t8.^6.844e-1;
t29 = t8.^4.187;
t30 = t8.^1.1444;
t31 = t8.^7.249;
t32 = t8-7.164e-1;
t33 = t8-7.204e-1;
t34 = t8-1.5445;
t35 = t8-1.3444;
t36 = t8-1.4517;
t37 = t32.^2;
t38 = t33.^2;
t39 = t34.^2;
t40 = t35.^2;
t41 = t36.^2;
t42 = t14.*(4.89e+2./1.0e+3);
t43 = t16.*(1.03e+2./1.0e+3);
t45 = t17.*(3.37e+2./2.0e+2);
t46 = t15.*2.506;
t50 = t18.*1.607;
t71 = rho.*t7.*t19.*5.012986845499098e-5;
t73 = t3.*t7.*t26.*9.43639666993474e-14;
t44 = -t42;
t47 = -t43;
t48 = -t45;
t49 = -t46;
t51 = -t50;
t52 = t37.*(1.71e+2./1.0e+3);
t53 = t40.*2.245e-1;
t55 = t38.*2.785e-1;
t58 = t39.*3.967e-1;
t59 = t41.*1.304e-1;
t54 = -t52;
t56 = -t53;
t57 = -t55;
t60 = -t58;
t61 = -t59;
t62 = t44+t56;
t63 = t48+t54;
t65 = t49+t57;
t67 = t47+t61;
t70 = t51+t60;
t64 = exp(t62);
t66 = exp(t63);
t68 = exp(t65);
t69 = exp(t67);
t72 = exp(t70);
et1 = t20.*4.52059+t25.*2.1101-t28.*6.93643+t71-t73+rho.*t24.*9.447562548362136e-5-rho.*t30.*1.729249419654372e-4+t3.*t4.*3.554762889834598e-13;
et2 = t7.*t19.*(-7.77414e-1)+t2.*t27.*1.633921676808176e-9+t22.*t64.*2.26312e-2+t21.*t72.*5.57346e-2-t31.*t68.*2.31752e-2;
et3 = rho.*t29.*t66.*(-2.730410110910498e-6)+t2.*t7.*t26.*4.390189186720438e-9+t2.*t23.*t69.*4.015042715686892e-10;
et4 = rho.*t31.*t68.*(rho.*3.231880319834924e-4-3.35804).*1.494402888831571e-6-rho.*t22.*t64.*(rho.*6.30642249161723e-5-1.52568e-1).*1.459324219757545e-6;
et5 = rho.*t21.*t72.*(rho.*2.072478720660304e-4-5.341668).*(-3.593925715759608e-6)+t2.*t29.*t66.*(rho.*2.17307196285788e-4-5.07522).*8.803230948254119e-11;
et6 = t3.*t23.*t69.*(rho.*1.328346659788496e-5-3.57616e-1).*(-8.630046246425269e-15);
et7 = t4.*6.258030493939e+1-t71+t73+log(-exp(t4.*(-5.309999999993605e+2))+1.0).*(2.02e+2./1.25e+2)-log(-exp(t4.*(-1.98899999999884e+3))+1.0).*(9.9e+1./1.25e+2);
et8 = log(-exp(t4.*(-6.858999999999336e+3))+1.0).*1.217+log(-exp(t4.*(-2.484000000001446e+3))+1.0).*(3.79e+2./5.0e+2)-log(-exp(t4.*(-7.51000000000887e+2))+1.0).*4.117e-1+log(t5)+log(t8).*(3.0./2.0);
et9 = rho.*t20.*2.915005158627805e-4+rho.*t25.*1.360652566417333e-4-rho.*t28.*4.472807583182873e-4+t2.*t24.*3.046028678218383e-9+t3.*t27.*3.5119974138255e-14;
et10 = t2.*t30.*(-5.575346336259904e-9)+t2.^2.*t4.*5.730530838655208e-18+t5.*(et1+et2+et3+et4+et5+et6)+rho.*t22.*t64.*1.459324219757545e-6+rho.*t21.*t72.*3.593925715759608e-6-rho.*t31.*t68.*1.494402888831571e-6;
et11 = t3.*t23.*t69.*8.630046246425269e-15-t2.*t29.*t66.*8.803230948254119e-11-4.579856474999999e-1;
g = T.*(et7+et8+et9+et10+et11).*8.314472;

== matlab function base_lib/F0001_panasonicCell/F0001_dynamicVoltage.m ==
  data: in1 input; dx output; T input; i input; V output
function [dx,V] = F0001_dynamicVoltage2(in1,T,i)
%BATTERYMODEL
%    [DX,V] = BATTERYMODEL(IN1,T,I)

%    This function was generated by the Symbolic Math Toolbox version 8.7.
%    02-Apr-2022 22:29:23

x1 = in1(1,:);
x2 = in1(2,:);
x3 = in1(3,:);
x4 = in1(4,:);
x5 = in1(5,:);
t2 = abs(i);
t3 = T.^2;
t5 = T.*1.191538469793427e+2;
t4 = t2.^2;
t6 = t2.*3.727678923610498e+2;
t7 = t5+t6+1.522023870656536e+3;
t8 = 1.0./t7;
et1 = T.*1.24826954009334e-4+t2.*4.819446179569201e-3;
et2 = t3.*(-1.270473422276427e-5)-t4.*4.61451648803152e-4;
et3 = T.*t2.*7.328585354340358e-5-3.630586079057569e-2;
et4 = T.*3.12067385023335e-5+t2.*1.2048615448923e-3;
et5 = t3.*(-3.176183555691067e-6)-t4.*1.15362912200788e-4;
et6 = T.*t2.*1.83214633858509e-5-9.076465197643922e-3;
et7 = T.*1.386966155659266e-5+t2.*5.354940199521335e-4;
et8 = t3.*(-1.411637135862696e-6)-t4.*5.127240542257244e-5;
et9 = T.*t2.*8.142872615933731e-6-4.033984532286187e-3;
et10 = T.*7.801684625583374e-6+t2.*3.012153862230751e-4;
et11 = t3.*(-7.940458889227668e-7)-t4.*2.8840728050197e-5;
et12 = T.*t2.*4.580365846462724e-6-2.26911629941098e-3;
et13 = T.*4.99307816037336e-6+t2.*1.927778471827681e-4;
et14 = t3.*(-5.081893689105708e-7)-t4.*1.845806595212608e-5;
et15 = T.*t2.*2.931434141736143e-6-1.452234431623028e-3;
dx = [i+(t8.*x1)./(et1+et2+et3);i+(t8.*x2)./(et4+et5+et6);i+(t8.*x3)./(et7+et8+et9);i+(t8.*x4)./(et10+et11+et12);i+(t8.*x5)./(et13+et14+et15)];
if nargout > 1
    et16 = T.*(-3.9634064763378e-3)-t2.*3.350735047934658e-3+t3.*6.415036047911208e-5+t4.*8.829330685388394e-5+T.*t2.*7.933830899953405e-5;
    et17 = 9.538952169556378e-2;
    V = t8.*x1+t8.*x2+t8.*x3+t8.*x4+t8.*x5+i.*(et16+et17);
end

== matlab function base_lib/F0005_h2Thermodynamics/F0005_helmholtz.m ==
  data: T input; a output; rho input
function a = F0005_helmholtz(T,rho)
%HELMHOLTZENERGY
%    A = HELMHOLTZENERGY(T,RHO)

%    This function was generated by the Symbolic Math Toolbox version 8.7.
%    04-Nov-2021 19:06:02

t2 = rho.^2;
t3 = rho.^3;
t4 = 1.0./T;
t5 = rho./1.5508e+4;
t6 = -t5;
t8 = t4.*3.3145e+1;
t7 = exp(t6);
et1 = t4.*6.258030493939e+1+log(-exp(t4.*(-5.309999999993605e+2))+1.0).*(2.02e+2./1.25e+2)-log(-exp(t4.*(-1.98899999999884e+3))+1.0).*(9.9e+1./1.25e+2);
et2 = log(-exp(t4.*(-6.858999999999336e+3))+1.0).*1.217+log(-exp(t4.*(-2.484000000001446e+3))+1.0).*(3.79e+2./5.0e+2)-log(-exp(t4.*(-7.51000000000887e+2))+1.0).*4.117e-1+log(t5)+log(t8).*(3.0./2.0);
et3 = rho.*t8.^(4.89e+2./1.0e+3).*2.915005158627805e-4+rho.*t8.^(9.89e+2./1.0e+3).*1.360652566417333e-4-rho.*t8.^6.844e-1.*4.472807583182873e-4+t2.^2.*t4.*5.730530838655208e-18;
et4 = t2.*t8.^(8.03e+2./1.0e+3).*3.046028678218383e-9+t3.*t8.^1.409.*3.5119974138255e-14-t2.*t8.^1.1444.*5.575346336259904e-9-rho.*t7.*t8.^(8.77e+2./5.0e+2).*5.012986845499098e-5;
et5 = t3.*t7.*t8.^1.311.*9.43639666993474e-14+rho.*t8.^5.646.*exp((t5-3.9e+1./2.5e+2).^2.*(-4.89e+2./1.0e+3)-(t8-1.3444).^2.*2.245e-1).*1.459324219757545e-6;
et6 = rho.*t8.^7.249.*exp((t5-6.7e+1./1.0e+2).^2.*(-2.506)-(t8-7.204e-1).^2.*2.785e-1).*(-1.494402888831571e-6);
et7 = rho.*t8.^2.986.*exp((t5-8.31e+2./5.0e+2).^2.*(-1.607)-(t8-1.5445).^2.*3.967e-1).*3.593925715759608e-6;
et8 = t2.*t8.^4.187.*exp((t5-7.53e+2./5.0e+2).^2.*(-3.37e+2./2.0e+2)-(t8-7.164e-1).^2.*(1.71e+2./1.0e+3)).*(-8.803230948254119e-11);
et9 = t3.*t8.^(7.91e+2./1.0e+3).*exp((t5-2.17e+2./1.25e+2).^2.*(-1.03e+2./1.0e+3)-(t8-1.4517).^2.*1.304e-1).*8.630046246425269e-15-1.4579856475;
a = T.*(et1+et2+et3+et4+et5+et6+et7+et8+et9).*8.314472;

== matlab function base_lib/F0005_h2Thermodynamics/F0005_pressure.m ==
  data: T input; p output; rho input
function p = F0005_pressure(T,rho)
%PRESSURE
%    P = PRESSURE(T,RHO)

%    This function was generated by the Symbolic Math Toolbox version 8.7.
%    04-Nov-2021 19:06:02

t2 = rho.^2;
t3 = rho.^3;
t4 = 1.0./T;
t5 = rho./1.5508e+4;
t6 = -t5;
t8 = t4.*3.3145e+1;
t9 = t5-3.9e+1./2.5e+2;
t10 = t5-6.7e+1./1.0e+2;
t11 = t5-2.17e+2./1.25e+2;
t12 = t5-7.53e+2./5.0e+2;
t13 = t5-8.31e+2./5.0e+2;
t7 = exp(t6);
t14 = t9.^2;
t15 = t10.^2;
t16 = t11.^2;
t17 = t12.^2;
t18 = t13.^2;
t19 = t8.^(8.77e+2./5.0e+2);
t20 = t8.^2.986;
t21 = t8.^5.646;
t22 = t8.^(7.91e+2./1.0e+3);
t23 = t8.^1.311;
t24 = t8.^4.187;
t25 = t8.^7.249;
t26 = t8-7.164e-1;
t27 = t8-7.204e-1;
t28 = t8-1.5445;
t29 = t8-1.3444;
t30 = t8-1.4517;
t31 = t26.^2;
t32 = t27.^2;
t33 = t28.^2;
t34 = t29.^2;
t35 = t30.^2;
t36 = t14.*(4.89e+2./1.0e+3);
t37 = t16.*(1.03e+2./1.0e+3);
t39 = t17.*(3.37e+2./2.0e+2);
t40 = t15.*2.506;
t44 = t18.*1.607;
t38 = -t36;
t41 = -t37;
t42 = -t39;
t43 = -t40;
t45 = -t44;
t46 = t31.*(1.71e+2./1.0e+3);
t47 = t34.*2.245e-1;
t49 = t32.*2.785e-1;
t52 = t33.*3.967e-1;
t53 = t35.*1.304e-1;
t48 = -t46;
t50 = -t47;
t51 = -t49;
t54 = -t52;
t55 = -t53;
t56 = t38+t50;
t57 = t42+t48;
t59 = t43+t51;
t61 = t41+t55;
t64 = t45+t54;
t58 = exp(t56);
t60 = exp(t57);
t62 = exp(t59);
t63 = exp(t61);
t65 = exp(t64);
et1 = t3.*t4.*3.554762889834598e-13-t7.*t19.*7.77414e-1+t21.*t58.*2.26312e-2+t20.*t65.*5.57346e-2-t25.*t62.*2.31752e-2;
et2 = rho.*t8.^(8.03e+2./1.0e+3).*9.447562548362136e-5-rho.*t8.^1.1444.*1.729249419654372e-4+t2.*t8.^1.409.*1.633921676808176e-9+t8.^(4.89e+2./1.0e+3).*4.52059;
et3 = t8.^(9.89e+2./1.0e+3).*2.1101-t8.^6.844e-1.*6.93643+rho.*t7.*t19.*5.012986845499098e-5-rho.*t24.*t60.*2.730410110910498e-6+t2.*t7.*t23.*4.390189186720438e-9;
et4 = t3.*t7.*t23.*(-9.43639666993474e-14)+t2.*t22.*t63.*4.015042715686892e-10+rho.*t25.*t62.*(rho.*3.231880319834924e-4-3.35804).*1.494402888831571e-6;
et5 = rho.*t21.*t58.*(rho.*6.30642249161723e-5-1.52568e-1).*(-1.459324219757545e-6)-rho.*t20.*t65.*(rho.*2.072478720660304e-4-5.341668).*3.593925715759608e-6;
et6 = t2.*t24.*t60.*(rho.*2.17307196285788e-4-5.07522).*8.803230948254119e-11-t3.*t22.*t63.*(rho.*1.328346659788496e-5-3.57616e-1).*8.630046246425269e-15;
p = T.*rho.*(t5.*(et1+et2+et3+et4+et5+et6)+1.0).*8.314472;

== matlab function base_lib/F0006_truckBenchmark/F0006_airDrag.m ==
  data: v input; Fa output; par parameter
function Fa = F0006_airDrag(v, par)
% inputs:
% v [m/s] - vehicle speed

% parameters:
rho_air = par.rho_air;
A_f     = par.A_f; % 10;
C_d     = par.C_d; % 0.5;

% output:
Fa = 1/2 * rho_air .* A_f .* C_d .* v.^2;
end

== matlab function base_lib/F0006_truckBenchmark/F0006_brakeForce.m ==
  data: brake input; Fb output; par parameter
function Fb = F0006_brakeForce(brake, par)
% inputs:
% brake [0,1] - brake signal

% parameters:
m    = par.m;
g    = 9.82;
gain = par.gain;

% output
Fb = min(min(max(brake,0),1) .* gain, m.*g);
end

== matlab function base_lib/F0006_truckBenchmark/F0006_gearBox.m ==
  data: Tq_in input; Tq_out output; w_out input; gear_ratio input; w_in output; par parameter
function [Tq_out, w_in] = F0006_gearBox(Tq_in, w_out, gear_ratio, par)
% parameters
fd_ratio = par.fd_ratio;
eta_gb   = par.eta_gb;

% combined drive ratio
gam = fd_ratio .* gear_ratio;

% torque on wheel
Tq_out = Tq_in .* gam .* eta_gb.^(sign(Tq_in));

% electric motor angular speed
w_in = w_out .* fd_ratio .* gear_ratio;

end

== matlab function base_lib/F0006_truckBenchmark/F0006_gravitationalForce.m ==
  data: alpha input; Fg output; par parameter
function Fg = F0006_gravitationalForce(alpha, par)
% inputs:
% alpha [rad] - road slope

% parameters:
m       = par.m;
g       = 9.82;

% output
Fg =   m .* g .* sin(alpha);
end

== matlab function base_lib/F0006_truckBenchmark/F0006_rollingResistance.m ==
  data: v input; Fr output; alpha input; par parameter
function Fr = F0006_rollingResistance(v, alpha, par)
% inputs:
% v     [m/s] - vehicle speed
% alpha [rad] - road slope

% parameters:
c_r0 = par.c_r0;
c_r1 = par.c_r1;
m    = par.m;
g    = 9.82;

% m/s -> km/h
v_k = v * 3.6;

% rolling resistance coefficient
c_r = c_r0 + c_r1 .* v_k.^2;

% output
Fr =  c_r .* m .* g .* cos(alpha);
end

== matlab function base_lib/F0007_ellipseCompressor/F0007_compressorEfficiency.m ==
  data: W_c input; eta_c output; p_us input; p_ds input; par parameter
function eta_c = F0007_compressorEfficiency(W_c, p_us, p_ds, par)

% parameters
eta_c_max = par.eta_c_max;
PiC_max   = par.PiC_max;
mco_max   = par.mco_max;
Q11       = par.Q11;
Q12       = par.Q12;
Q22       = par.Q22;

% pressure ratio
PiC = p_ds./p_us;

% Model 8.5, Compressor Efficiency
% Equation (8.41-42)
eta_c = ...
eta_c_max - ...
    ( (PiC - 1).^(1/2) - (PiC_max - 1).^(1/2)) .* ...
    ( Q12.*W_c - Q12.*mco_max + (Q22.*abs(PiC - 1))./(PiC - 1).^(1/2) - (Q22.*abs(PiC_max - 1))./(PiC_max - 1).^(1/2)) - ...
    (W_c - mco_max) .* ...
    (Q11.*(W_c - mco_max) + Q12.*(conj((PiC - 1).^(1/2)) - ...
    conj((PiC_max - 1).^(1/2))));

end

== matlab function base_lib/F0007_ellipseCompressor/F0007_compressorFlow.m ==
  data: p_us input; W_c output; p_ds input; T_us input; w_c input; par parameter
function W_c = F0007_compressorFlow(p_us, p_ds, T_us, w_c, par)

% parameters
k1 = par.k1;
k2 = par.k2;

% constants
g   = 1.4;
R   = 280;
cp  = g*R/(g-1);
D   = 56e-3;

% ideal gas law for density
rho01 = p_us ./ (R.*T_us);

% Pressure Ratio (Pi)
Pi = p_ds./p_us;

% Energy Coefficient (Psi)
% Equation (8.46)
Psi = cp .* T_us .* ( Pi.^( (g-1)/g ) - 1 ) ./ ( w_c.^2 .* D.^2 );

% Flow Coefficient (Phi)
% Equation (8.52)
Psi = max(min(Psi,k2),1e-3);
Phi = k1 .* sqrt(1 - (Psi ./ k2).^2 );

% Compressor mass flow
% Equation (8.53)
W_c = Phi .* rho01 .* w_c .* D.^3;

end

== matlab function base_lib/F0007_ellipseCompressor/F0007_compressorPower.m ==
  data: W_c input; P_c output; T_us input; T_ds input
function P_c = F0007_compressorPower(W_c, T_us, T_ds)

% model constants
g   = 1.4;
R   = 280;
cp  = g*R/(g-1);

% compressor work
% eq. 8.5d
P_c = cp .* W_c .* (T_ds - T_us);

end

== matlab function base_lib/F0007_ellipseCompressor/F0007_compressorTemperature.m ==
  data: p_us input; T_ds output; p_ds input; T_us input; eta_c input
function T_ds = F0007_compressorTemperature(p_us, p_ds, T_us, eta_c)

% model constants
g = 1.4;

% pressure ratio
PiC = p_ds./p_us;

% compressor out temperature (adiabatic)
T_ds = T_us + T_us ./ eta_c .* ( PiC.^((g-1)/g)  - 1  );

end

== matlab function base_lib/F0001_panasonicCell/F0001_cellCapacity.m ==
  data: T input; Q0 output
function Q0 = cellCapacity(T)
% Fit to cycle data from
% Li-Ion Battery Model Performance for Automotive Drive
% Cycles with Current Pulse and EIS Parameterization
% Kolmeyer et al, 
% 978-1-5090-3953-1/$31.00 ©2017 IEEE

% parameters
a0 = 2.5718;
a1 = 0.0307;
a2 = -0.0006;

Q0 = a0 + a1.*T + a2 .*T^2;
end

== matlab function base_lib/F0007_ellipseCompressor/F0007_multicomponentFlow.m ==
  data: p_us input; W_split output; W_tot input; par parameter
function W_split = F0007_multicomponentFlow(p_us, W_tot, par)
% output size
W = zeros(3,1);

% total pressure
p_tot = sum(p_us);

% partial pressures
p_r  = p_us(1);
p_v  = p_us(2);
p_N2 = p_us(3);

% mole fractions
x_r   = p_r  ./ p_tot;
x_v   = p_v  ./ p_tot;
x_N2  = p_N2 ./ p_tot;

% average mass
M_avg = sum([x_r, x_v, x_N2] .* [par.M_r, par.M_H2O, par.M_N2]);

% mole fraction to mass fraction
w_r   = x_r  .* par.M_r   ./ M_avg;
w_v   = x_v  .* par.M_H2O ./ M_avg;
w_N2  = x_N2 .* par.M_N2  ./ M_avg;

% outlet species convective mass flow
W_split = W_tot .* [w_r; w_v; w_N2];

end

== matlab function base_lib/F0007_ellipseCompressor/F0007_shaftTorqueBalance.m ==
  data: Tq_em input; dw_c output; Tq_c input; w_c input
function dw_c = F0007_shaftTorqueBalance(Tq_em, Tq_c, w_c)

% constants
J_c = 1e-5;
c   = 1e-6;

% shaft friction
Mf = c .* w_c;

% turbo shaft dynamics
% Model 8.3
dw_c = 1/J_c .* ( Tq_em - Tq_c - Mf);

end

== matlab function base_lib/F0008_throttle/F0008_throttleFlow.m ==
  data: alpha input; W_th output; p_us input; p_ds input; T_us input; par parameter
function W_th = F0008_throttleFlow(alpha, p_us, p_ds, T_us, par)

% model parameters
a0 = par.a0;
a1 = par.a1;
a2 = par.a2;

% Parameters
cp_j = par.cp_j; % [J/kgK]  - Specific heats
M_j  = par.M_j;  % [kg/mol] - Molar masses
R_j  = par.R_j;  % [J/kgK]  - Specific gas constant


% total pressures
p_us_tot = sum(p_us);
p_ds_tot = sum(p_ds);

% Mole fractions
x_us     = p_us ./ p_us_tot;

% Average molar mass
M_avg = sum(x_us .* M_j);

% Mole fraction to mass fraction
w_us = x_us .* M_j ./ M_avg;

% Mixture gas constant & specific heat
R_m  = sum(w_us .* R_j);
cp_m = sum(w_us .* cp_j);

% specific heat ratio
cv_m = cp_m - R_m;
g    = cp_m ./ cv_m;

% effective area
Aeff = a0 + a1.*alpha + a2 .* alpha.^2;

% pressure ratio
Pi = p_ds_tot./p_us_tot;

% Pi_lim
Pi_lim = max( Pi, ...
             (2./(g+1)).^( g./(g-1) ) ...
             );

% Psi
Psi = sqrt( ...
            2.*g./(g-1) .*  ...
            ( Pi_lim.^(2./g) - Pi_lim.^((g+1)./g) ) ...
           );


       
       
       
       
% mass flow
W_th = p_us_tot./sqrt(R_m.*T_us) .* Aeff .* Psi;

end
